simulink model "volume_adapt"  (R2024b)
settings: Solver=FixedStepDiscrete  StartTime=0.0  StopTime=inf  FixedStep=dt  RelTol=1e-3
values from neighbouring files (symbols this model uses):
  vBlockParams = struct    [pressure_control.m]
undefined symbols (not defined in the file or in its folder): disfilt, dspblkCoreblockFVToolHelper, dta, gcbh
libraries: simulink x3, subsignallib x2
settings Model: SimulationMode=external  ExtModeEnableFloating=off  ExtModeTrigDuration=100000  Creator=pro  LastModifiedBy=af49v
settings SolverCC: ConcurrentTasks=on  AlgebraicLoopSolver=TrustRegion  PositivePriorityOrder=on  AutoInsertRateTranBlk=on
settings DataIOCC: MaxDataPoints=500  SaveOutput=off  DSMLogging=off  SaveTime=off  ReturnWorkspaceOutputs=off
settings OptimizationCC: BlockReduction=off  OptimizeBlockIOStorage=off  EnhancedBackFolding=on  PassReuseOutputArgsThreshold=0  MaxStackSize=64  OptimizeBlockOrder=speed  DifferentSizesBufferReuse=on
settings DebuggingCC: AlgebraicLoopMsg=error  TasksWithSamePriorityMsg=none  IntegerOverflowMsg=error  ParameterUnderflowMsg=error  ParameterTunabilityLossMsg=error  UnconnectedInputMsg=warning  UnconnectedOutputMsg=warning  UnconnectedLineMsg=warning  AllowSymbolicDim=off  NonBusSignalsTreatedAsBus=error  SFInvalidInputDataAccessInChartInitDiag=error
settings HardwareCC: ProdBitPerLong=64  ProdLongLongMode=on  ProdHWDeviceType=Intel->x86-64 (Linux 64)  HardwareBoardFeatureSet=SoCBlockset
settings ModelReferenceCC: EnableRefExpFcnMdlSchedulingChecks=on
settings SFSimCC: MATLABDynamicMemAlloc=off
settings RTWCC: Description=Speedgoat Real-Time Target Machine  SystemTargetFile=speedgoat.tlc  TemplateMakefile=slrealtime_default_tmf  RTWVerbose=off  Toolchain=Simulink Real-Time Toolchain  BuildConfiguration=Faster Runs  CodeExecutionProfiling=on  TargetLang=C++  GPUComputeCapability=3.5  DLArmComputeVersion=19.05
settings CodeAppCC: ForceParamTrailComments=on  OperatorAnnotations=on
settings SimulinkRealTimeTargetCC: InstructionSetFMA=off  LogToMDFFile=off

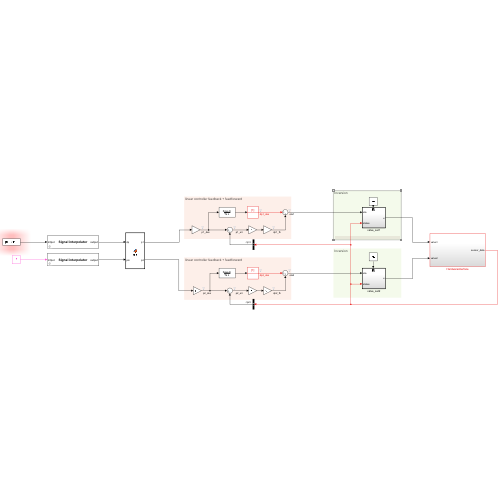
[thumbnail: Simulink's stored preview of the top-level diagram]
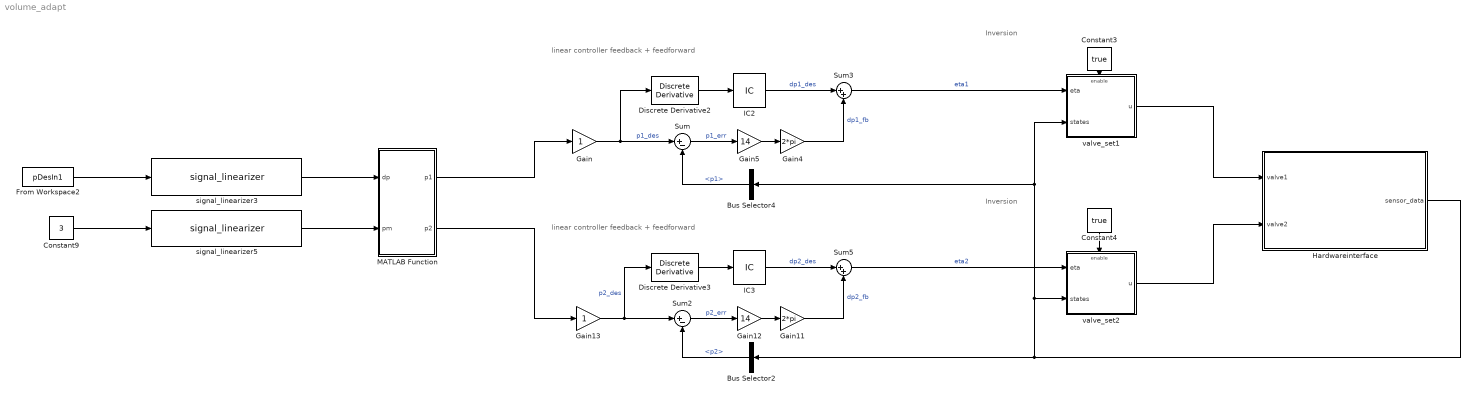
== system volume_adapt ==
  note: linear controller feedback + feedforward
  note: linear controller feedback + feedforward
  note: Inversion
  note: Inversion
  Bus Selector2 : BusSelector  OutputSignals=p2
  Bus Selector4 : BusSelector  OutputSignals=p1
  Constant3 : Constant  Value=true
  Constant4 : Constant  Value=true
  Constant9 : Constant  Value=3
  Discrete Derivative2 : simulink/Discrete/Discrete Derivative  gainval=1.0  ICPrevScaledInput=0.0  OutMin=[]  OutMax=[]  OutDataType=fixdt(1, 16)  OutScaling=2^-10  DoSatur=off
  Discrete Derivative3 : simulink/Discrete/Discrete Derivative  gainval=1.0  ICPrevScaledInput=0.0  OutMin=[]  OutMax=[]  OutDataType=fixdt(1, 16)  OutScaling=2^-10  DoSatur=off
  From Workspace2 : FromWorkspace  VariableName=pDesIn1  SampleTime=dta
  Gain : Gain
  Gain11 : Gain  Gain=2*pi
  Gain12 : Gain  Gain=14
  Gain13 : Gain
  Gain4 : Gain  Gain=2*pi
  Gain5 : Gain  Gain=14
  Hardwareinterface : Subsystem
  IC2 : InitialCondition
  IC3 : InitialCondition
  MATLAB Function : MATLAB Function  TreatAsAtomicUnit=on
  Sum : Sum  Inputs=|+-
  Sum2 : Sum  Inputs=|+-
  Sum3 : Sum  Inputs=|++
  Sum5 : Sum  Inputs=|++
  signal_linearizer3 : subsignallib/signal_linearizer  param_low=dta  param_high=dt  es_filt_enabled=off  es_ts=10
      settings: SourceProductName=Signals
  signal_linearizer5 : subsignallib/signal_linearizer  param_low=2  param_high=dt  es_filt_enabled=off  es_ts=10
      settings: SourceProductName=Signals
  valve_set1 : Subsystem
  valve_set2 : Subsystem
  wires:
  signal_linearizer3/1 -> MATLAB Function/1(dp)
  signal_linearizer5/1 -> MATLAB Function/2(pm)
  From Workspace2/1 -> signal_linearizer3/1
  MATLAB Function/1(p1) -> Gain/1
  Constant9/1 -> signal_linearizer5/1
  MATLAB Function/2(p2) -> Gain13/1
  Hardwareinterface/1(sensor_data) -> Bus Selector2/1, valve_set1/2(states), Bus Selector4/1, valve_set2/2(states)
  valve_set2/1(u) -> Hardwareinterface/2(valve2)
  Constant4/1 -> valve_set2/Enable
  Constant3/1 -> valve_set1/Enable
  valve_set1/1(u) -> Hardwareinterface/1(valve1)
  Sum5/1 -> valve_set2/1(eta)  "eta2"
  Sum3/1 -> valve_set1/1(eta)  "eta1"
  Gain13/1 -> Discrete Derivative3/1, Sum2/1  "p2_des"
  Discrete Derivative3/1 -> IC3/1
  Gain11/1 -> Sum5/2  "dp2_fb"
  Gain12/1 -> Gain11/1
  Sum2/1 -> Gain12/1  "p2_err"
  IC3/1 -> Sum5/1  "dp2_des"
  Bus Selector2/1 -> Sum2/2  "<p2>"
  Bus Selector4/1 -> Sum/2  "<p1>"
  Gain/1 -> Sum/1, Discrete Derivative2/1  "p1_des"
  Discrete Derivative2/1 -> IC2/1
  Gain5/1 -> Gain4/1
  IC2/1 -> Sum3/1  "dp1_des"
  Sum/1 -> Gain5/1  "p1_err"
  Gain4/1 -> Sum3/2  "dp1_fb"

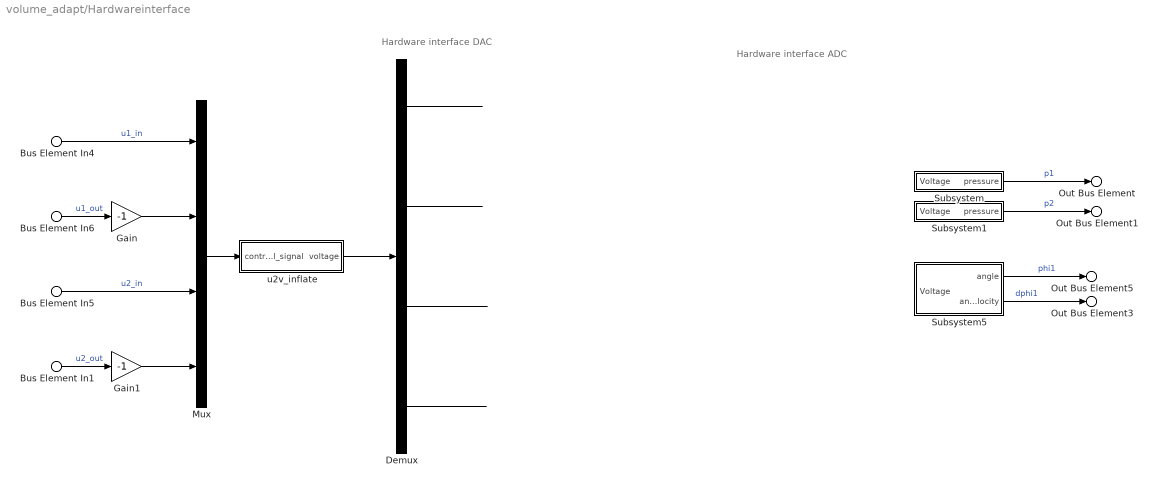
== system volume_adapt/Hardwareinterface ==
  note: Hardware interface ADC
  note: Hardware interface DAC
  Bus Element In4 : Inport  PortName=valve1  Element=u_in
  Bus Element In6 : Inport  PortName=valve1  Element=u_out
  Bus Element In5 : Inport  Port=2  PortName=valve2  Element=u_in
  Bus Element In1 : Inport  Port=2  PortName=valve2  Element=u_out
  Demux : Demux
  Gain : Gain  Gain=-1
  Gain1 : Gain  Gain=-1
  Mux : Mux
  Subsystem : Subsystem
  Subsystem1 : Subsystem
  Subsystem5 : Subsystem
  u2v_inflate : Subsystem
  Out Bus Element : Outport  PortName=sensor_data  Element=p1
  Out Bus Element1 : Outport  PortName=sensor_data  Element=p2
  Out Bus Element5 : Outport  PortName=sensor_data  Element=phi1
  Out Bus Element3 : Outport  PortName=sensor_data  Element=dphi1
  wires:
  Subsystem/1(pressure) -> Out Bus Element/1  "p1"
  ? -> Subsystem/1(Voltage)
  ? -> Subsystem1/1(Voltage)
  Subsystem1/1(pressure) -> Out Bus Element1/1  "p2"
  Bus Element In4/1 -> Mux/1  "u1_in"
  ? -> Subsystem5/1(Voltage)
  Subsystem5/1(angle) -> Out Bus Element5/1  "phi1"
  Bus Element In6/1 -> Gain/1  "u1_out"
  Gain/1 -> Mux/2
  Bus Element In5/1 -> Mux/3  "u2_in"
  Bus Element In1/1 -> Gain1/1  "u2_out"
  Gain1/1 -> Mux/4
  Subsystem5/2(angle velocity) -> Out Bus Element3/1  "dphi1"
  Mux/1 -> u2v_inflate/1(control_signal)
  u2v_inflate/1(voltage) -> Demux/1
  Demux/1 -> ?
  Demux/2 -> ?
  Demux/3 -> ?
  Demux/4 -> ?

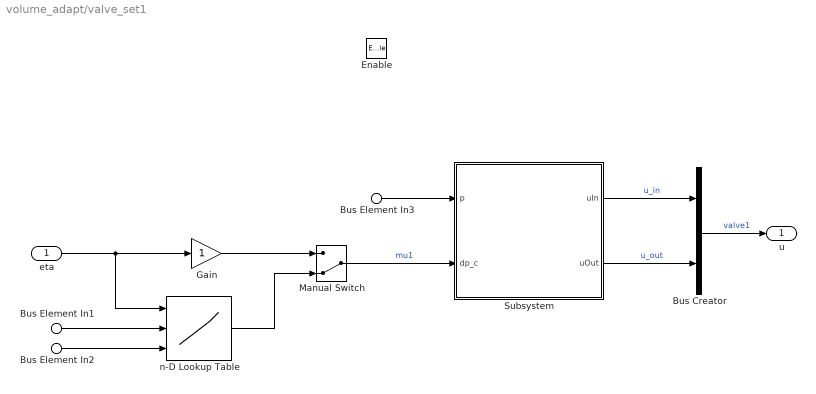
== system volume_adapt/valve_set1 ==
  eta : Inport
  Bus Element In3 : Inport  Port=2  PortName=states  Element=p1
  Bus Element In1 : Inport  Port=2  PortName=states  Element=phi1
  Bus Element In2 : Inport  Port=2  PortName=states  Element=dphi1
  Enable : EnablePort
  Bus Creator : BusCreator  Inputs=2
  Gain : Gain
  Manual Switch : ManualSwitch  CurrentSetting=0
  Subsystem : Subsystem
      mask Display:
      | port_label('input', 1, 'p')
      | port_label('input', 2, 'dp_c')
      | 
      | port_label('output', 1, 'u_in')
      | port_label('output', 2, 'u_out')
      | 
      | disp('{\bf\fontsize{12}Valve function \xi(p, dp)}', 'texmode','on');
  n-D Lookup Table : Lookup_n-D  NumberOfTableDimensions=3  BreakpointsForDimension1=vBlockParams.valveblock1.eta  BreakpointsForDimension2=vBlockParams.valveblock1.phi  BreakpointsForDimension3=vBlockParams.valveblock1.dphi  Table=vBlockParams.valveblock1.muPred  InternalRulePriority=Speed  RndMeth=Simplest
      settings: InputPortMap=u0,u1,u2
  u : Outport  OutputWhenDisabled=reset  InitialOutput=0
  wires:
  Bus Element In3/1 -> Subsystem/1(p)
  Manual Switch/1 -> Subsystem/2(dp_c)  "mu1"
  Subsystem/1(uIn) -> Bus Creator/1  "u_in"
  eta/1 -> n-D Lookup Table/1, Gain/1
  n-D Lookup Table/1 -> Manual Switch/2
  Bus Creator/1 -> u/1  "valve1"
  Subsystem/2(uOut) -> Bus Creator/2  "u_out"
  Bus Element In1/1 -> n-D Lookup Table/2
  Gain/1 -> Manual Switch/1
  Bus Element In2/1 -> n-D Lookup Table/3

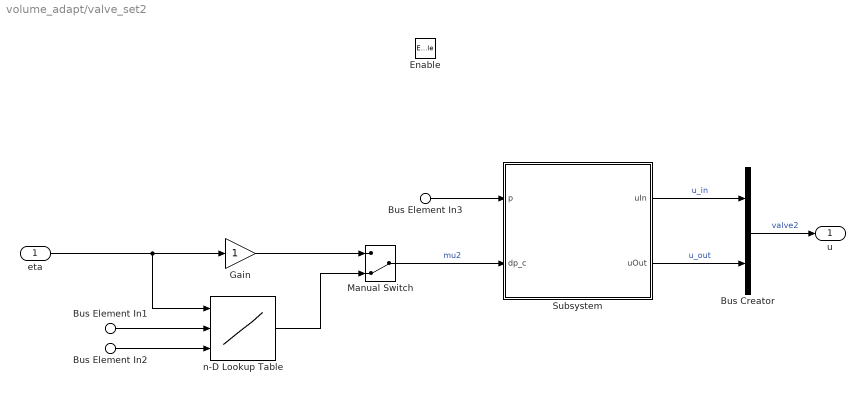
== system volume_adapt/valve_set2 ==
  eta : Inport
  Bus Element In3 : Inport  Port=2  PortName=states  Element=p2
  Bus Element In1 : Inport  Port=2  PortName=states  Element=phi1
  Bus Element In2 : Inport  Port=2  PortName=states  Element=dphi1
  Enable : EnablePort
  Bus Creator : BusCreator  Inputs=2
  Gain : Gain
  Manual Switch : ManualSwitch  CurrentSetting=0
  Subsystem : Subsystem
      mask Display:
      | port_label('input', 1, 'p')
      | port_label('input', 2, 'dp_c')
      | 
      | port_label('output', 1, 'u_in')
      | port_label('output', 2, 'u_out')
      | 
      | disp('{\bf\fontsize{12}Valve function \xi(p, dp)}', 'texmode','on');
  n-D Lookup Table : Lookup_n-D  NumberOfTableDimensions=3  BreakpointsForDimension1=vBlockParams.valveblock2.eta  BreakpointsForDimension2=vBlockParams.valveblock2.phi  BreakpointsForDimension3=vBlockParams.valveblock2.dphi  Table=vBlockParams.valveblock2.muPred  InternalRulePriority=Speed  RndMeth=Simplest
      settings: InputPortMap=u0,u1,u2
  u : Outport  OutputWhenDisabled=reset  InitialOutput=0
  wires:
  Subsystem/2(uOut) -> Bus Creator/2  "u_out"
  Bus Creator/1 -> u/1  "valve2"
  n-D Lookup Table/1 -> Manual Switch/2
  eta/1 -> Gain/1, n-D Lookup Table/1
  Subsystem/1(uIn) -> Bus Creator/1  "u_in"
  Manual Switch/1 -> Subsystem/2(dp_c)  "mu2"
  Bus Element In3/1 -> Subsystem/1(p)
  Gain/1 -> Manual Switch/1
  Bus Element In1/1 -> n-D Lookup Table/2
  Bus Element In2/1 -> n-D Lookup Table/3

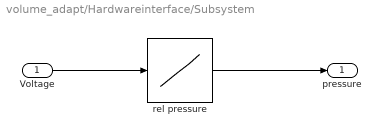
== system volume_adapt/Hardwareinterface/Subsystem ==
  Voltage : Inport
  rel pressure : Lookup_n-D  NumberOfTableDimensions=1  BreakpointsForDimension1=[0 10]  Table=[0 10]  InternalRulePriority=Speed  RndMeth=Simplest
  pressure : Outport  VectorParamsAs1DForOutWhenUnconnected=off
  wires:
  Voltage/1 -> rel pressure/1
  rel pressure/1 -> pressure/1

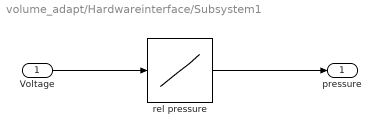
== system volume_adapt/Hardwareinterface/Subsystem1 ==
  Voltage : Inport
  rel pressure : Lookup_n-D  NumberOfTableDimensions=1  BreakpointsForDimension1=[0 10]  Table=[0 10]  InternalRulePriority=Speed  RndMeth=Simplest
  pressure : Outport  VectorParamsAs1DForOutWhenUnconnected=off
  wires:
  Voltage/1 -> rel pressure/1
  rel pressure/1 -> pressure/1

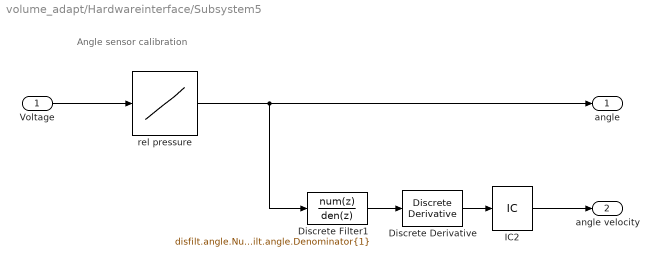
== system volume_adapt/Hardwareinterface/Subsystem5 ==
  note: Angle sensor calibration
  Voltage : Inport
  Discrete Derivative : simulink/Discrete/Discrete Derivative  gainval=1.0  ICPrevScaledInput=0.0  OutMin=[]  OutMax=[]  OutDataType=fixdt(1, 16)  OutScaling=2^-10  DoSatur=off
  Discrete Filter1 : DiscreteFilter  LoadFcn=dspblkCoreblockFVToolHelper(gcbh,'load');  Numerator=disfilt.angle.Numerator{1}  Denominator=disfilt.angle.Denominator{1}
      settings: CopyFcn=dspblkCoreblockFVToolHelper(gcbh,'copy');  DeleteFcn=dspblkCoreblockFVToolHelper(gcbh,'close');  ModelCloseFcn=dspblkCoreblockFVToolHelper(gcbh,'close');  PreSaveFcn=dspblkCoreblockFVToolHelper(gcbh,'presave');  PostSaveFcn=dspblkCoreblockFVToolHelper(gcbh,'postsave');  CloseFcn=dspblkCoreblockFVToolHelper(gcbh,'close');
  IC2 : InitialCondition
  rel pressure : Lookup_n-D  NumberOfTableDimensions=1  BreakpointsForDimension1=[2.167 3.14]  Table=[0.7854 -0.7854]  InternalRulePriority=Speed  RndMeth=Simplest
  angle : Outport  VectorParamsAs1DForOutWhenUnconnected=off
  angle velocity : Outport  Port=2  VectorParamsAs1DForOutWhenUnconnected=off
  wires:
  Discrete Derivative/1 -> IC2/1
  IC2/1 -> angle velocity/1
  rel pressure/1 -> angle/1, Discrete Filter1/1
  Discrete Filter1/1 -> Discrete Derivative/1
  Voltage/1 -> rel pressure/1

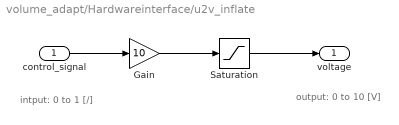
== system volume_adapt/Hardwareinterface/u2v_inflate ==
  note: intput: 0 to 1 [/]
  note: output: 0 to 10 [V]
  control_signal : Inport
  Gain : Gain  Gain=10
  Saturation : Saturate  UpperLimit=10  LowerLimit=0
  voltage : Outport  VectorParamsAs1DForOutWhenUnconnected=off
  wires:
  Gain/1 -> Saturation/1
  control_signal/1 -> Gain/1
  Saturation/1 -> voltage/1

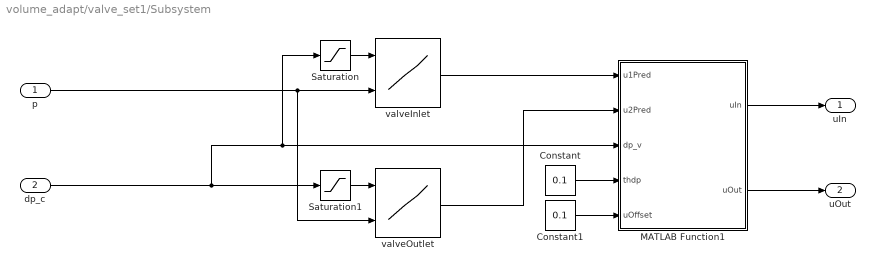
== system volume_adapt/valve_set1/Subsystem ==
  p : Inport
  dp_c : Inport  Port=2
  Constant : Constant  Value=0.1
  Constant1 : Constant  Value=0.1
  MATLAB Function1 : MATLAB Function  TreatAsAtomicUnit=on
  Saturation : Saturate  UpperLimit=inf  LowerLimit=0
  Saturation1 : Saturate  UpperLimit=0  LowerLimit=-inf
  valveInlet : Lookup_n-D  BreakpointsForDimension1=vBlockParams.valveblock1.dpField.pos  BreakpointsForDimension2=vBlockParams.valveblock1.pField  Table=vBlockParams.valveblock1.uPred.pos  ExtrapMethod=Clip  InternalRulePriority=Speed  RndMeth=Simplest
      settings: InputPortMap=u0,u1
  valveOutlet : Lookup_n-D  BreakpointsForDimension1=vBlockParams.valveblock1.dpField.neg  BreakpointsForDimension2=vBlockParams.valveblock1.pField  Table=vBlockParams.valveblock1.uPred.neg  ExtrapMethod=Clip  InternalRulePriority=Speed  RndMeth=Simplest
      settings: InputPortMap=u0,u1
  uIn : Outport
  uOut : Outport  Port=2
  wires:
  Saturation1/1 -> valveOutlet/1
  valveInlet/1 -> MATLAB Function1/1(u1Pred)
  dp_c/1 -> Saturation1/1, Saturation/1, MATLAB Function1/3(dp_v)
  Constant/1 -> MATLAB Function1/4(thdp)
  Constant1/1 -> MATLAB Function1/5(uOffset)
  valveOutlet/1 -> MATLAB Function1/2(u2Pred)
  MATLAB Function1/2(uOut) -> uOut/1
  MATLAB Function1/1(uIn) -> uIn/1
  Saturation/1 -> valveInlet/1
  p/1 -> valveOutlet/2, valveInlet/2

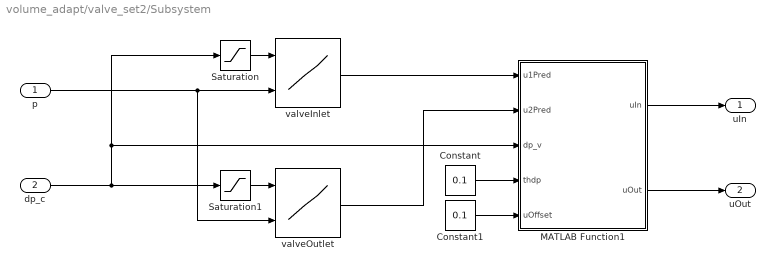
== system volume_adapt/valve_set2/Subsystem ==
  p : Inport
  dp_c : Inport  Port=2
  Constant : Constant  Value=0.1
  Constant1 : Constant  Value=0.1
  MATLAB Function1 : MATLAB Function  TreatAsAtomicUnit=on
  Saturation : Saturate  UpperLimit=inf  LowerLimit=0
  Saturation1 : Saturate  UpperLimit=0  LowerLimit=-inf
  valveInlet : Lookup_n-D  BreakpointsForDimension1=vBlockParams.valveblock2.dpField.pos  BreakpointsForDimension2=vBlockParams.valveblock2.pField  Table=vBlockParams.valveblock2.uPred.pos  ExtrapMethod=Clip  InternalRulePriority=Speed  RndMeth=Simplest
      settings: InputPortMap=u0,u1
  valveOutlet : Lookup_n-D  BreakpointsForDimension1=vBlockParams.valveblock2.dpField.neg  BreakpointsForDimension2=vBlockParams.valveblock2.pField  Table=vBlockParams.valveblock2.uPred.neg  ExtrapMethod=Clip  InternalRulePriority=Speed  RndMeth=Simplest
      settings: InputPortMap=u0,u1
  uIn : Outport
  uOut : Outport  Port=2
  wires:
  dp_c/1 -> Saturation/1, MATLAB Function1/3(dp_v), Saturation1/1
  MATLAB Function1/1(uIn) -> uIn/1
  MATLAB Function1/2(uOut) -> uOut/1
  Constant1/1 -> MATLAB Function1/5(uOffset)
  Constant/1 -> MATLAB Function1/4(thdp)
  Saturation/1 -> valveInlet/1
  p/1 -> valveInlet/2, valveOutlet/2
  Saturation1/1 -> valveOutlet/1
  valveInlet/1 -> MATLAB Function1/1(u1Pred)
  valveOutlet/1 -> MATLAB Function1/2(u2Pred)

== matlab function volume_adapt/MATLAB Function ==
  data: dp input; p1 output; pm input; p2 output
function [p1, p2] = fcn(dp, pm)
p1 = pm+1/2*dp;
p2 = pm-1/2*dp;

== matlab function volume_adapt/valve_set1/Subsystem/MATLAB Function1 ==
  data: uIn output; u1Pred input; u2Pred input; uOut output; dp_v input; thdp input; uOffset input
function [uIn, uOut] = fcn(u1Pred, u2Pred, dp_v, thdp, uOffset)
uIn = u1Pred - (dp_v < thdp)*uOffset;
uOut = u2Pred + (dp_v > -thdp)*uOffset;

== matlab function volume_adapt/valve_set2/Subsystem/MATLAB Function1 ==
  data: uIn output; u1Pred input; u2Pred input; uOut output; dp_v input; thdp input; uOffset input
function [uIn, uOut] = fcn(u1Pred, u2Pred, dp_v, thdp, uOffset)
uIn = u1Pred - (dp_v < thdp)*uOffset;
uOut = u2Pred + (dp_v > -thdp)*uOffset;
